simulink model "Example_HBridge_Simulation"  (R2014a)
settings: Solver=ode45  StartTime=0.0  StopTime=10.0  RelTol=1e-3
libraries: powerlib x9
settings Model: Creator=Humayun Gazi  LastModifiedBy=Humayun Gazi

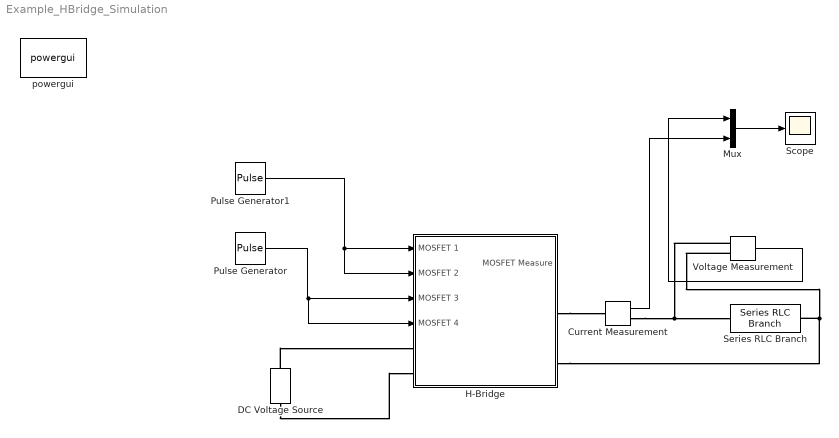
== system Example_HBridge_Simulation ==
  Current Measurement : powerlib/Measurements/Current Measurement  PhasorSimulation=off  OutputType=Complex  PSBequivalent=0
  DC Voltage Source : powerlib/Electrical Sources/DC Voltage Source  Amplitude=100  Measurements=None
  "H-Bridge " : Subsystem
  Mux : Mux  Inputs=2
  Pulse Generator : DiscretePulseGenerator  PulseType=Time based  Period=20e-3  PulseWidth=50  PhaseDelay=10e-3
  Pulse Generator1 : DiscretePulseGenerator  PulseType=Time based  Period=20e-3  PulseWidth=50
  Scope : Scope
      settings: YMin=-200  YMax=200
  Series RLC Branch : powerlib/Elements/Series RLC Branch  LConnTagsString=__new0  RConnTagsString=__new0  BranchType=RL  Resistance=1  Inductance=5e-3  SetiL0=off  InitialCurrent=0  Capacitance=1e-6  Setx0=off  InitialVoltage=0  Measurements=None
  Voltage Measurement : powerlib/Measurements/Voltage Measurement  PhasorSimulation=off  OutputType=Complex  PSBequivalent=0
  powergui : powerlib/powergui  Priority=1  SimulationMode=Continuous  SolverType=Tustin  SampleTime=50e-6  frequency=60  SPID=off  DisableSnubberDevices=off  DisableRonSwitches=off  DisableVfSwitches=off  SwTol=0  Interpol=off  DisplayEquations=off  Ts=0  methode=off  frequencyindice=0  Pbase=100e6  ErrMax=1e-4  Iterations=50  UnitsV=kV  UnitsW=MW  FunctionMessages=off  echomessages=off  HookPort=off  EnableUseOfTLC=off  x0status=blocks  RestoreLinks=warning  ResistiveCurrentMeasurement=off  Frange=[0:2:500]  Ylog=off  Xlog=on  ShowGrid=off  save=off  variable=ZData  structure=0  ZoomFFT=off  StartTime=0.0  cycles=1  DisplayStyle=1  fundamental=60  FreqAxis=off  MaxFrequency=1000  frequencyindicesteady=1  RmsSteady=1  display=off
  wires:
  Pulse Generator1/1 -> "H-Bridge "/2(MOSFET 2), "H-Bridge "/1(MOSFET 1)
  Pulse Generator/1 -> "H-Bridge "/4(MOSFET 4), "H-Bridge "/3(MOSFET 3)
  Voltage Measurement/1 -> Mux/1
  Current Measurement/1 -> Mux/2
  Mux/1 -> Scope/1
  connections:
  DC Voltage Source/RConn1 -- "H-Bridge "/LConn1
  DC Voltage Source/LConn1 -- "H-Bridge "/LConn2
  "H-Bridge "/RConn1 -- Current Measurement/LConn1
  Current Measurement/RConn1 -- Voltage Measurement/LConn1 -- Series RLC Branch/LConn1
  Voltage Measurement/LConn2 -- "H-Bridge "/RConn2 -- Series RLC Branch/RConn1

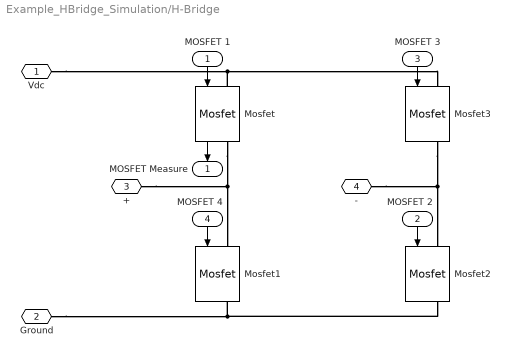
== system Example_HBridge_Simulation/H-Bridge  ==
  MOSFET 1 : Inport
  MOSFET 2 : Inport  Port=2
  MOSFET 3 : Inport  Port=3
  MOSFET 4 : Inport  Port=4
  Mosfet{,1..3} (4 alike) : powerlib/Power Electronics/Mosfet  Ron=0.1  Lon=0  Rd=0.01  Vfd=0  IC=0  Rs=1e5  Cs=inf  Measurements=on
  Vdc : PMIOPort  Port=1  Side=Left
  Ground : PMIOPort  Port=2  Side=Left
  + : PMIOPort  Port=3  Side=Right
  - : PMIOPort  Port=4  Side=Right
  MOSFET Measure : Outport
  wires:
  MOSFET 1/1 -> Mosfet/1
  MOSFET 3/1 -> Mosfet3/1
  MOSFET 2/1 -> Mosfet2/1
  Mosfet/1 -> MOSFET Measure/1
  MOSFET 4/1 -> Mosfet1/1
  connections:
  Mosfet/LConn1 -- Vdc/RConn1 -- Mosfet3/LConn1
  Mosfet3/RConn1 -- -/RConn1 -- Mosfet2/LConn1
  Mosfet2/RConn1 -- Ground/RConn1 -- Mosfet1/RConn1
  Mosfet/RConn1 -- +/RConn1 -- Mosfet1/LConn1
